simulink model "simpleVector"  (R2022b)
settings: Solver=VariableStepAuto  StartTime=0.0  StopTime=10.0  RelTol=1e-3  EnableMultiTasking=on
settings Model: Creator=jrivitus  LastModifiedBy=bensweet
settings SolverCC: AlgebraicLoopSolver=TrustRegion
settings DataIOCC: LimitDataPoints=on  SaveFormat=Array  ReturnWorkspaceOutputs=off
settings OptimizationCC: ExpressionDepthLimit=2147483647  InitFltsAndDblsToZero=on  LifeSpan=inf
settings DebuggingCC: UnconnectedInputMsg=warning  UnconnectedOutputMsg=warning  UnconnectedLineMsg=warning  PregeneratedLibrarySubsystemCodeDiagnostic=none  SFMachineParentedDataDiag=warning
settings HardwareCC: ProdBitPerPointer=32  ProdBitPerSizeT=32  ProdBitPerPtrDiffT=32  ProdLargestAtomicFloat=None  ProdIntDivRoundTo=Undefined  ProdEndianess=Unspecified  ProdWordSize=32  ProdHWDeviceType=32-bit Generic
settings ModelReferenceCC: EnableRefExpFcnMdlSchedulingChecks=on  PropagateSignalLabelsOutOfModel=off
settings SFSimCC: SimUseLocalCustomCode=off
settings RTWCC: RTWUseLocalCustomCode=off  DLArmComputeVersion=19.05
settings CodeAppCC: StateflowObjectComments=on
settings GRTTargetCC: TargetLangStandard=C89/C90 (ANSI)  CombineOutputUpdateFcns=off  GRTInterface=on
settings ConfigComp: CovMetricSettings=dw  CovSaveCumulativeToWorkspaceVar=on  CovSaveSingleToWorkspaceVar=on  CovExternalEMLEnable=off  CovSFcnEnable=off

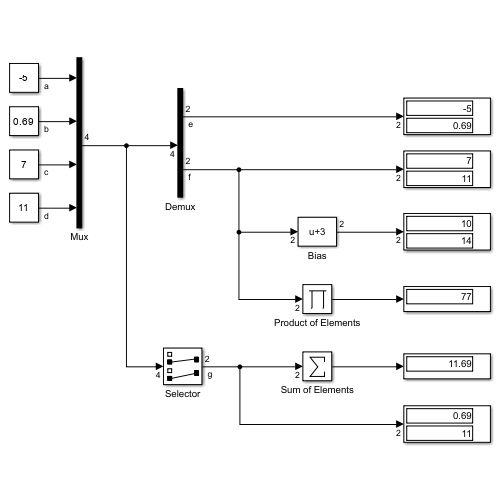
[thumbnail: Simulink's stored preview of the top-level diagram]
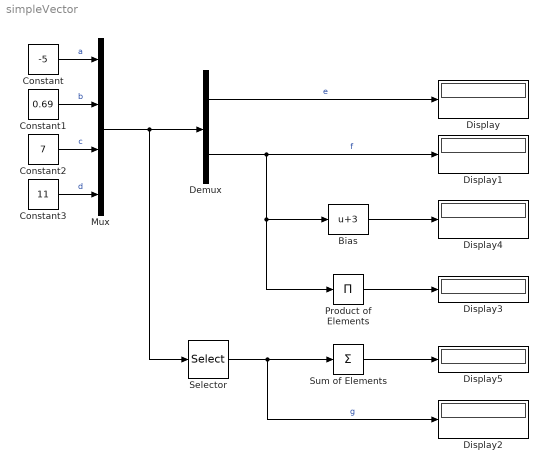
== system simpleVector ==
  Bias : Bias  Bias=3  SaturateOnIntegerOverflow=off
  Constant : Constant  Value=-5
  Constant1 : Constant  Value=0.69
  Constant2 : Constant  Value=7
  Constant3 : Constant  Value=11
  Demux : Demux  Outputs=2
  Display{,1..5} (6 alike) : Display
  Mux : Mux
  Product of Elements : Product  Inputs=*
  Selector : Selector  InputPortWidth=4  IndexOptions=Index vector (dialog)  Indices=[2 4]  OutputSizes=1
  Sum of Elements : Sum  Inputs=+
  wires:
  Constant/1 -> Mux/1  "a"
  Constant1/1 -> Mux/2  "b"
  Constant2/1 -> Mux/3  "c"
  Constant3/1 -> Mux/4  "d"
  Mux/1 -> Demux/1, Selector/1
  Selector/1 -> Sum of Elements/1, Display2/1  "g"
  Demux/1 -> Display/1  "e"
  Demux/2 -> Display1/1, Product of Elements/1, Bias/1  "f"
  Product of Elements/1 -> Display3/1
  Bias/1 -> Display4/1
  Sum of Elements/1 -> Display5/1
